simulink model "SteerControlUnit_8"  (R2014a)
settings: Solver=ode15s  StartTime=0.0  StopTime=10.0  RelTol=1e-3
undefined symbols (not defined in the file): sigbuilder_block
libraries: fl_lib x11, sh_lib x9, nesl_utility x7
Description:
  | Copyright 2014 The MathWorks, Inc.
settings Model: Creator=wnursilo  LastModifiedBy=smiller
settings DataIOCC: SignalLoggingSaveFormat=ModelDataLogs
settings OptimizationCC: ExpressionDepthLimit=2147483647  InitFltsAndDblsToZero=on
settings DebuggingCC: UnderspecifiedInitializationDetection=Classic  FcnCallInpInsideContextMsg=UseLocalSettings  StateNameClashWarn=warning
settings GRTTargetCC: CombineOutputUpdateFcns=off  GRTInterface=on

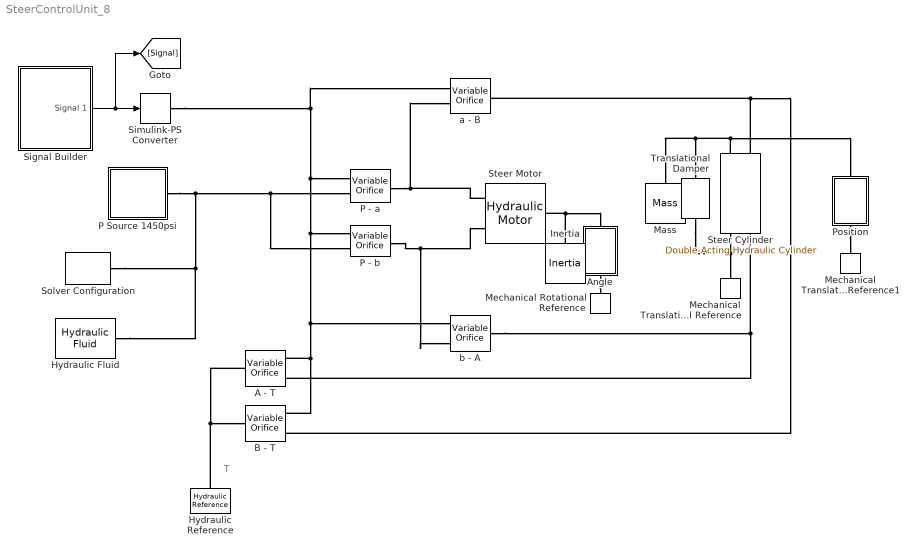
== system SteerControlUnit_8 ==
  note: T
  A - T : sh_lib/Orifices/Variable Orifice  mdl_type=1  area_max=5e-05 m^2  opening_max=6 mm  opening_tab="[  -0.002 0 0.002 0.005 0.015 ] m"  area_tab="[  1e-09 2.0352e-07 4.0736e-05 0.00011438 0.00034356 ] m^2"  pressure_tab="[  -1e+07 -5e+06 -2e+06 2e+06 5e+06 1e+07 ] Pa"  flow_rate_tab="[  -1e-07 -7.0711e-08 -4.4721e-08 4.4721e-08 7.0711e-08 1e-07 ; -2.0352e-05 -1.4391e-05 -9.1017e-06 9.1017e-06 1.4391e-05 2.0352e-05 ; -0.0040736 -0.0028805 -0.0018218 0.0018218 0.0028805 0.0040736 ; -0.011438 -0.0080879 -0.0051152 0.0051152 0.0080879 0.011438 ; -0.034356 -0.024293 -0.015364 0.015364 0.024293 0.034356 ; ] m^3/s"  interp_method=1  extrap_method=1  or=1  C_d=0.7  x_0=-3 mm  Re_cr=12  A_leak=1e-12 m^2  cst=100 N  x_or=1
  Angle : Subsystem
      settings: OpenFcn=|
      | open_system([gcb '/angle']);
      | close_system(gcs);                    hh=findobj(allchild(0),'name','angle');
      | ha=findobj(hh(1),'type','axes');
      | set(get(ha,'title'),'string',get(gcbh,'name'));
      | clear hh ha;
      mask Display:
      | plot([0,1],[1,1]);
      | plot([1,1],[1,2]);
      | plot([1,0],[2,2]);
      | plot([0,0],[2,1]);
      | patch([0 0 0],[2.4 2.4 2.4],[0 0 0]);
      | patch([1 1 1],[0 0 0],[0 0 0]);
      | port_label('RConn', 1,'|');
      | port_label('LConn', 1,'+')
  B - T : sh_lib/Orifices/Variable Orifice  mdl_type=1  area_max=5e-05 m^2  opening_max=6 mm  opening_tab="[  -0.002 0 0.002 0.005 0.015 ] m"  area_tab="[  1e-09 2.0352e-07 4.0736e-05 0.00011438 0.00034356 ] m^2"  pressure_tab="[  -1e+07 -5e+06 -2e+06 2e+06 5e+06 1e+07 ] Pa"  flow_rate_tab="[  -1e-07 -7.0711e-08 -4.4721e-08 4.4721e-08 7.0711e-08 1e-07 ; -2.0352e-05 -1.4391e-05 -9.1017e-06 9.1017e-06 1.4391e-05 2.0352e-05 ; -0.0040736 -0.0028805 -0.0018218 0.0018218 0.0028805 0.0040736 ; -0.011438 -0.0080879 -0.0051152 0.0051152 0.0080879 0.011438 ; -0.034356 -0.024293 -0.015364 0.015364 0.024293 0.034356 ; ] m^3/s"  interp_method=1  extrap_method=1  or=2  C_d=0.7  x_0=-3 mm  Re_cr=12  A_leak=1e-12 m^2  cst=100 N  x_or=1
  Hydraulic Fluid : sh_lib/Hydraulic Utilities/Hydraulic Fluid  DataSource=1  SelFluid=5  SysTemp=60 c  TrapAir=0.005  ViscDerFactor=1  range_error=2
  Hydraulic Reference : fl_lib/Hydraulic/Hydraulic Elements/Hydraulic Reference
  Inertia : fl_lib/Mechanical/Rotational Elements/Inertia  inertia=0.001 kg*m^2  w_specify=on  w_priority=High  w=0 rad/s  t_specify=off  t_priority=High  t=0 N*m
  Mass : fl_lib/Mechanical/Translational Elements/Mass  mass=10 kg  v_specify=on  v_priority=High  v=0 m/s  f_specify=off  f_priority=High  f=0 N
  Mechanical Rotational Reference : fl_lib/Mechanical/Rotational Elements/Mechanical Rotational Reference
  Mechanical Translational Reference : fl_lib/Mechanical/Translational Elements/Mechanical Translational Reference
  Mechanical Translational Reference1 : fl_lib/Mechanical/Translational Elements/Mechanical Translational Reference
  P - a : sh_lib/Orifices/Variable Orifice  mdl_type=1  area_max=5e-05 m^2  opening_max=6 mm  opening_tab="[  -0.002 0 0.002 0.005 0.015 ] m"  area_tab="[  1e-09 2.0352e-07 4.0736e-05 0.00011438 0.00034356 ] m^2"  pressure_tab="[  -1e+07 -5e+06 -2e+06 2e+06 5e+06 1e+07 ] Pa"  flow_rate_tab="[  -1e-07 -7.0711e-08 -4.4721e-08 4.4721e-08 7.0711e-08 1e-07 ; -2.0352e-05 -1.4391e-05 -9.1017e-06 9.1017e-06 1.4391e-05 2.0352e-05 ; -0.0040736 -0.0028805 -0.0018218 0.0018218 0.0028805 0.0040736 ; -0.011438 -0.0080879 -0.0051152 0.0051152 0.0080879 0.011438 ; -0.034356 -0.024293 -0.015364 0.015364 0.024293 0.034356 ; ] m^3/s"  interp_method=1  extrap_method=1  or=2  C_d=0.7  x_0=-3 mm  Re_cr=12  A_leak=1e-12 m^2  cst=100 N  x_or=1
  P - b : sh_lib/Orifices/Variable Orifice  mdl_type=1  area_max=5e-05 m^2  opening_max=6 mm  opening_tab="[  -0.002 0 0.002 0.005 0.015 ] m"  area_tab="[  1e-09 2.0352e-07 4.0736e-05 0.00011438 0.00034356 ] m^2"  pressure_tab="[  -1e+07 -5e+06 -2e+06 2e+06 5e+06 1e+07 ] Pa"  flow_rate_tab="[  -1e-07 -7.0711e-08 -4.4721e-08 4.4721e-08 7.0711e-08 1e-07 ; -2.0352e-05 -1.4391e-05 -9.1017e-06 9.1017e-06 1.4391e-05 2.0352e-05 ; -0.0040736 -0.0028805 -0.0018218 0.0018218 0.0028805 0.0040736 ; -0.011438 -0.0080879 -0.0051152 0.0051152 0.0080879 0.011438 ; -0.034356 -0.024293 -0.015364 0.015364 0.024293 0.034356 ; ] m^3/s"  interp_method=1  extrap_method=1  or=1  C_d=0.7  x_0=-3 mm  Re_cr=12  A_leak=1e-12 m^2  cst=100 N  x_or=1
  P Source 1450psi : Subsystem
  Position : Subsystem
      settings: OpenFcn=|
      | open_system([gcb '/position']);
      | close_system(gcs);                    hh=findobj(allchild(0),'name','position');
      | ha=findobj(hh(1),'type','axes');
      | set(get(ha,'title'),'string',get(gcbh,'name'));
      | clear hh ha;
      mask Display:
      | plot([0,1],[1,1]);
      | plot([1,1],[1,2]);
      | plot([1,0],[2,2]);
      | plot([0,0],[2,1]);
      | patch([0 0 0],[2.4 2.4 2.4],[0 0 0]);
      | patch([1 1 1],[0 0 0],[0 0 0]);
      | port_label('RConn', 1,'|');
      | port_label('LConn', 1,'+')
  Signal Builder : Subsystem  Tag=STV Subsys  LoadFcn=sigbuilder_block('load');  StartFcn=sigbuilder_block('start');  StopFcn=sigbuilder_block('stop');  ClipboardFcn=sigbuilder_block('clipboard');  mask(Sigbuilder block){}
      mask help: Sigbuilder GUI
      mask init:
      | if ~strcmp(get_param(bdroot(gcbh),'SimulationStatus'),'stopped') tuvar = sigbuilder_block('maskInit'); end
      settings: CopyFcn=sigbuilder_block('copy');  DeleteFcn=sigbuilder_block('delete');  ModelCloseFcn=sigbuilder_block('modelClose');  PreSaveFcn=sigbuilder_block('preSave');  PauseFcn=sigbuilder_block('pause')  ContinueFcn=sigbuilder_block('continue')  NameChangeFcn=sigbuilder_block('namechange');  OpenFcn=sigbuilder_block('open',[140.25 72 550.5 399.75 ]);  CloseFcn=sigbuilder_block('close');
      mask Display: plot(0,0,100,100,[10,10,40,40,10],[80,20,20,80,80],[40,10],[50,50], [40,27,10],[65,72,56],[40,25,25,10],[28,28,43,43]);
  Simulink-PS Converter : nesl_utility/Simulink-PS Converter  PhysicalDomain=network_engine_domain  SubClassName=ps_input  LeftPortType=input  RightPortType=output  PseudoPeriodic=off  Frequencies=[]  NoiseDistribution=none  NoiseParameters=[]  Unit=mm  AffineConversion=off  InputFiltering=off  SimscapeFilterOrder=1  InputFilterTimeConstant=.001  UdotUserProvided=0
  Solver Configuration : nesl_utility/Solver Configuration  PhysicalDomain=network_engine_domain  SubClassName=solver  LeftPortType=input  RightPortType=generic  Accelerate=off  Tones=[]  Harmonics=[]  SimulateNoise=off  Profile=off  UseLocalSampling=off  EnableSwitchedLinearOptims=on  FrequencyDomain=off  UseCCode=off  RelTol=0.001  AbsTol=1e-06  MinStep=1e-09  ToWorkspace=off  DoDC=off  ResidualTolerance=1e-9  UseLocalSolver=off  LocalSolverChoice=NE_BACKWARD_EULER_ADVANCER  LocalSolverSampleTime=.001  DoFixedCost=off  MaxNonlinIter=12  MaxModeIter=2  LinearAlgebra=Sparse  DelaysMemoryBudget=1024  AutomaticFiltering=on  FilteringTimeConstant=0.001
  Steer Cylinder : sh_lib/Hydraulic Cylinders/Double-Acting Hydraulic Cylinder  area_A=0.25*pi*(3.25^2-2.5^2) in^2  area_B=0.25*pi*(3.25^2-2.5^2) in^2  stroke=6.38 in  init_pos=6.38/2 in  dead_vol_A=1e-04 m^3  dead_vol_B=1e-04 m^3  init_pressure_A=0 Pa  init_pressure_B=0 Pa  k_sh=1.4  stiff=1e+06 N/m  D=150 N/(m/s)  or=2  or_sign=1
  Steer Motor : sh_lib/Pumps and Motors/Hydraulic Motor  D=5e-06 m^3/rad  efficiency_vol=0.92  efficiency_tot=0.8  pr_nominal=1e+07 Pa  w_nominal=188 rad/s  visc_nominal=18 cSt  dens_nominal=900 kg/m^3  k_leak=1e-11 m^3/s/Pa  efficiency_mech=0.7
  Translational Damper : fl_lib/Mechanical/Translational Elements/Translational Damper  D=1000 N/(m/s)  v_specify=off  v_priority=High  v=0 m/s  f_specify=off  f_priority=High  f=0 N
  a - B : sh_lib/Orifices/Variable Orifice  mdl_type=1  area_max=5e-05 m^2  opening_max=6 mm  opening_tab="[  -0.002 0 0.002 0.005 0.015 ] m"  area_tab="[  1e-09 2.0352e-07 4.0736e-05 0.00011438 0.00034356 ] m^2"  pressure_tab="[  -1e+07 -5e+06 -2e+06 2e+06 5e+06 1e+07 ] Pa"  flow_rate_tab="[  -1e-07 -7.0711e-08 -4.4721e-08 4.4721e-08 7.0711e-08 1e-07 ; -2.0352e-05 -1.4391e-05 -9.1017e-06 9.1017e-06 1.4391e-05 2.0352e-05 ; -0.0040736 -0.0028805 -0.0018218 0.0018218 0.0028805 0.0040736 ; -0.011438 -0.0080879 -0.0051152 0.0051152 0.0080879 0.011438 ; -0.034356 -0.024293 -0.015364 0.015364 0.024293 0.034356 ; ] m^3/s"  interp_method=1  extrap_method=1  or=1  C_d=0.7  x_0=-3 mm  Re_cr=12  A_leak=1e-12 m^2  cst=100 N  x_or=1
  b - A : sh_lib/Orifices/Variable Orifice  mdl_type=1  area_max=5e-05 m^2  opening_max=6 mm  opening_tab="[  -0.002 0 0.002 0.005 0.015 ] m"  area_tab="[  1e-09 2.0352e-07 4.0736e-05 0.00011438 0.00034356 ] m^2"  pressure_tab="[  -1e+07 -5e+06 -2e+06 2e+06 5e+06 1e+07 ] Pa"  flow_rate_tab="[  -1e-07 -7.0711e-08 -4.4721e-08 4.4721e-08 7.0711e-08 1e-07 ; -2.0352e-05 -1.4391e-05 -9.1017e-06 9.1017e-06 1.4391e-05 2.0352e-05 ; -0.0040736 -0.0028805 -0.0018218 0.0018218 0.0028805 0.0040736 ; -0.011438 -0.0080879 -0.0051152 0.0051152 0.0080879 0.011438 ; -0.034356 -0.024293 -0.015364 0.015364 0.024293 0.034356 ; ] m^3/s"  interp_method=1  extrap_method=1  or=2  C_d=0.7  x_0=-3 mm  Re_cr=12  A_leak=1e-12 m^2  cst=100 N  x_or=1
  wires:
  Signal Builder/1(Signal 1) -> Simulink-PS Converter/1, [Signal]
  connections:
  P Source 1450psi/LConn1 -- Solver Configuration/RConn1 -- Hydraulic Fluid/RConn1 -- P - a/LConn2 -- P - b/LConn2
  Hydraulic Reference/LConn1 -- B - T/RConn1 -- A - T/RConn1
  Steer Cylinder/RConn1 -- Translational Damper/LConn1 -- Mass/LConn1 -- Position/LConn1
  Steer Motor/RConn1 -- Inertia/LConn1 -- Angle/LConn1
  Angle/RConn1 -- Mechanical Rotational Reference/LConn1
  P - b/RConn1 -- Steer Motor/LConn2 -- b - A/LConn2
  Steer Motor/LConn1 -- a - B/LConn2 -- P - a/RConn1
  Steer Cylinder/LConn1 -- Mechanical Translational Reference/LConn1 -- Translational Damper/RConn1
  Steer Cylinder/RConn2 -- a - B/RConn1 -- B - T/LConn2
  b - A/RConn1 -- Steer Cylinder/LConn2 -- A - T/LConn2
  P - a/LConn1 -- Simulink-PS Converter/RConn1 -- a - B/LConn1 -- P - b/LConn1 -- b - A/LConn1 -- A - T/LConn1 -- B - T/LConn1
  Position/RConn1 -- Mechanical Translational Reference1/LConn1

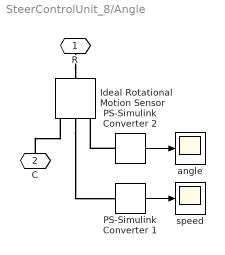
== system SteerControlUnit_8/Angle ==
  Ideal Rotational Motion Sensor : fl_lib/Mechanical/Mechanical Sensors/Ideal Rotational Motion Sensor  offset=0 rad
  PS-Simulink Converter 1 : nesl_utility/PS-Simulink Converter  PhysicalDomain=network_engine_domain  SubClassName=ps_output  LeftPortType=input  RightPortType=output  PseudoPeriodic=off  Frequencies=[]  Unit=1  AffineConversion=off
  PS-Simulink Converter 2 : nesl_utility/PS-Simulink Converter  PhysicalDomain=network_engine_domain  SubClassName=ps_output  LeftPortType=input  RightPortType=output  PseudoPeriodic=off  Frequencies=[]  Unit=1  AffineConversion=off
  angle : Scope
      settings: TimeRange=1  YMin=0  YMax=1  SaveName=ScopeData3
  speed : Scope
      settings: TimeRange=10  YMin=0  YMax=0.1  SaveName=ScopeData2
  R : PMIOPort  Port=1  Side=Left
  C : PMIOPort  Port=2  Side=Right
  wires:
  PS-Simulink Converter 1/1 -> speed/1
  PS-Simulink Converter 2/1 -> angle/1
  connections:
  Ideal Rotational Motion Sensor/RConn2 -- PS-Simulink Converter 1/LConn1
  PS-Simulink Converter 2/LConn1 -- Ideal Rotational Motion Sensor/RConn3
  R/RConn1 -- Ideal Rotational Motion Sensor/LConn1
  C/RConn1 -- Ideal Rotational Motion Sensor/RConn1

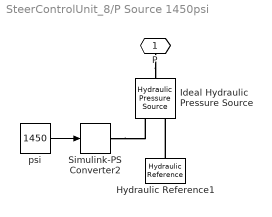
== system SteerControlUnit_8/P Source 1450psi ==
  Hydraulic Reference1 : fl_lib/Hydraulic/Hydraulic Elements/Hydraulic Reference
  Ideal Hydraulic Pressure Source : fl_lib/Hydraulic/Hydraulic Sources/Hydraulic Pressure Source
  Simulink-PS Converter2 : nesl_utility/Simulink-PS Converter  PhysicalDomain=network_engine_domain  SubClassName=ps_input  LeftPortType=input  RightPortType=output  PseudoPeriodic=off  Frequencies=[]  NoiseDistribution=none  NoiseParameters=[]  Unit=psi  AffineConversion=off  InputFiltering=off  SimscapeFilterOrder=1  InputFilterTimeConstant=.001  UdotUserProvided=0
  psi : Constant  Value=1450
  P : PMIOPort  Port=1  Side=Left
  wires:
  psi/1 -> Simulink-PS Converter2/1
  connections:
  Hydraulic Reference1/LConn1 -- Ideal Hydraulic Pressure Source/RConn2
  Simulink-PS Converter2/RConn1 -- Ideal Hydraulic Pressure Source/RConn1
  P/RConn1 -- Ideal Hydraulic Pressure Source/LConn1

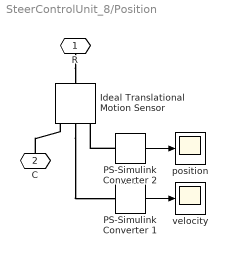
== system SteerControlUnit_8/Position ==
  Ideal Translational Motion Sensor : fl_lib/Mechanical/Mechanical Sensors/Ideal Translational Motion Sensor  offset=0 in
  PS-Simulink Converter 1 : nesl_utility/PS-Simulink Converter  PhysicalDomain=network_engine_domain  SubClassName=ps_output  LeftPortType=input  RightPortType=output  PseudoPeriodic=off  Frequencies=[]  Unit=1  AffineConversion=off
  PS-Simulink Converter 2 : nesl_utility/PS-Simulink Converter  PhysicalDomain=network_engine_domain  SubClassName=ps_output  LeftPortType=input  RightPortType=output  PseudoPeriodic=off  Frequencies=[]  Unit=in  AffineConversion=off
  position : Scope
      settings: TimeRange=1  YMin=7.23985  YMax=7.2406  SaveName=ScopeData3
  velocity : Scope
      settings: TimeRange=10  YMin=0  YMax=0.1  SaveName=ScopeData2
  R : PMIOPort  Port=1  Side=Left
  C : PMIOPort  Port=2  Side=Right
  wires:
  PS-Simulink Converter 2/1 -> position/1
  PS-Simulink Converter 1/1 -> velocity/1
  connections:
  PS-Simulink Converter 2/LConn1 -- Ideal Translational Motion Sensor/RConn3
  C/RConn1 -- Ideal Translational Motion Sensor/RConn1
  R/RConn1 -- Ideal Translational Motion Sensor/LConn1
  Ideal Translational Motion Sensor/RConn2 -- PS-Simulink Converter 1/LConn1

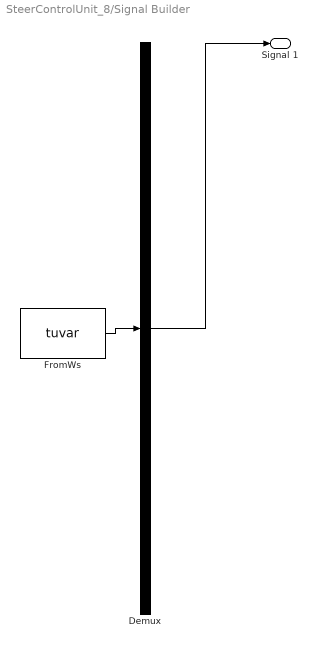
== system SteerControlUnit_8/Signal Builder ==
  Demux : Demux  Tag=STV Demux  Outputs=1
  FromWs : FromWorkspace  Tag=STV FromWs  VariableName=tuvar  SampleTime=0
      SigBuilderData=|
      | common.afterFinalStr = 'Extrapolate'
      | common.sampleTime = 0
      | dataSet.timeRange = [0 10]
      | dataSet.name = 'Group 1'
      | sbobj.Name = 'Signal Builder'
      | sbobj.Groups.Name = 'Group 1'
      | sbobj.Groups.Signals.Name = 'Signal 1'
      | sbobj.Groups.Signals.XData = [0 1 1.5 4.5 5 5.5 6 9 9.5 10]
      | sbobj.Groups.Signals.YData = [0 0 9 9 0 0 -9 -9 0 0]
  Signal 1 : Outport  Tag=STV Outport
  wires:
  Demux/1 -> Signal 1/1
  FromWs/1 -> Demux/1
